simulink model "fuzzylogicMPPTmodified"  (R2024a)
settings: Solver=VariableStepAuto  StartTime=0.0  StopTime=20  RelTol=1e-3
undefined symbols (not defined in the file): Acid, Lead
libraries: spsSeriesRLCBranchLib x8, spsDiodeLib x4, spsBatteryLib x2, spsMosfetLib x2, spsPVArrayLib x2, fuzblock x1, spsPWMGeneratorDCDCLib x1, simulink x1, spsVoltageMeasurementLib x1, sps_lib x1
settings Model: Creator=Lenovo  LastModifiedBy=Lenovo

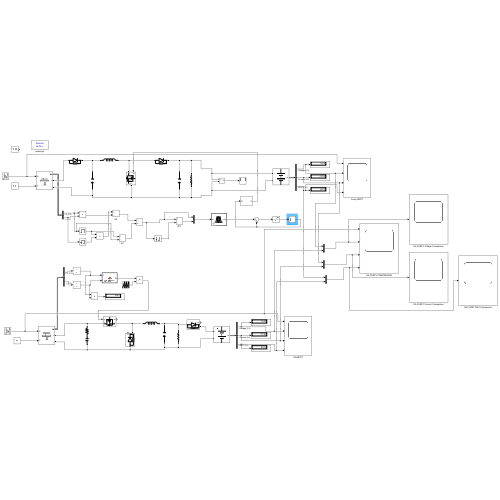
[thumbnail: Simulink's stored preview of the top-level diagram]
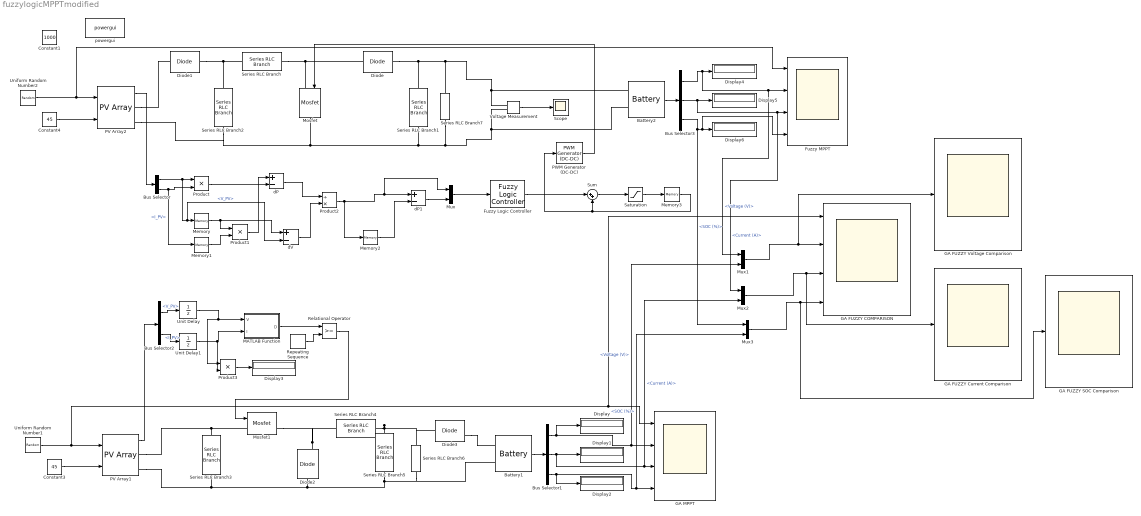
== system fuzzylogicMPPTmodified ==
  Battery1 : spsBatteryLib/Battery  BatType=Lead-Acid  ShowTempParam=off  ThermalPreset=no  ShowAgeParam=off  NomV=12  NomQ=40  SOC=60  Batt_Tr=0.1  PresetModel=on  MaxQ=41.6667  MinV=9  FullV=13.0658  Dis_rate=8  R=0.003  Normal_OP=12.4111  expZone="[12.2171     0.133333]"  current=[6.5 13 32.5]  Units=Time  Tci=20  NomT=20  T2=-30  MaxQ2=4.8  FullV2=7.1  Normal_OP2=5.655  expZone2="[6.58           1]"  Rca=0.6  ti=2000  Dp=0  Neq0=0  Tsim=1e6  Ta1=25  Qeol=5.4*0.9  Reol=0.013333*1.2  Char_age=[2.3478, 3]  Dis_age=[2.3478, 10]  N1=1500  N2=10500  N3=1000  N4=1400  Ta2=45  N5=950
  Battery2 : spsBatteryLib/Battery  BatType=Lead-Acid  ShowTempParam=off  ThermalPreset=no  ShowAgeParam=off  NomV=12  NomQ=40  SOC=60  Batt_Tr=0.1  PresetModel=on  MaxQ=41.6667  MinV=9  FullV=13.0658  Dis_rate=8  R=0.003  Normal_OP=12.4111  expZone="[12.2171     0.133333]"  current=[6.5 13 32.5]  Units=Time  Tci=20  NomT=20  T2=-30  MaxQ2=4.8  FullV2=7.1  Normal_OP2=5.655  expZone2="[6.58           1]"  Rca=0.6  ti=2000  Dp=0  Neq0=0  Tsim=1e6  Ta1=25  Qeol=5.4*0.9  Reol=0.013333*1.2  Char_age=[2.3478, 3]  Dis_age=[2.3478, 10]  N1=1500  N2=10500  N3=1000  N4=1400  Ta2=45  N5=950
  Bus Selector : BusSelector  OutputSignals=V_PV,I_PV
  Bus Selector1 : BusSelector  OutputSignals=Voltage (V),Current (A),SOC (%)
  Bus Selector2 : BusSelector  OutputSignals=V_PV,I_PV
  Bus Selector3 : BusSelector  OutputSignals=Voltage (V),Current (A),SOC (%)
  Constant1 : Constant  Value=1000
  Constant3 : Constant  Value=45
  Constant4 : Constant  Value=45
  Diode : spsDiodeLib/Diode  Ron=0.001  Lon=0  Vf=0.8  IC=0  UseSnubber=0  Rs=500  Cs=250e-9  Measurements=off
  Diode1 : spsDiodeLib/Diode  Ron=0.001  Lon=0  Vf=0.8  IC=0  UseSnubber=0  Rs=500  Cs=250e-9  Measurements=off
  Diode2 : spsDiodeLib/Diode  Ron=0.001  Lon=0  Vf=0.8  IC=0  UseSnubber=0  Rs=500  Cs=250e-9  Measurements=on
  Diode3 : spsDiodeLib/Diode  Ron=0.001  Lon=0  Vf=0.3  IC=0  UseSnubber=0  Rs=500  Cs=250e-9  Measurements=on
  Display{,1..6} (7 alike) : Display
  Fuzzy Logic Controller : fuzblock/Fuzzy Logic  Controller  FIS='pomppt.fis'  OutputSampleNumber=101  DataType=double  FuzzifiedInputs=off  RuleFiringStrengths=off  RuleOutputs=off  AggregatedOutputs=off  SimulateUsing=Interpreted execution  OutOfRangeInputValueMessage=warning  NoRuleFiredMessage=warning  EmptyOutputFuzzySetMessage=warning
  Fuzzy MPPT : Scope  NumInputPorts=4
  GA FUZZY COMPARISON : Scope  NumInputPorts=4
  GA FUZZY Current Comparison : Scope
  GA FUZZY SOC Comparison : Scope
  GA FUZZY Voltage Comparison : Scope
  GA MPPT : Scope  NumInputPorts=4
  MATLAB Function : MATLAB Function  TreatAsAtomicUnit=on
  Memory{,1..3} (4 alike) : Memory
  Mosfet : spsMosfetLib/Mosfet  Ron=0.1  Lon=0  Rd=0.01  Vfd=0  IC=0  Rs=1e5  Cs=inf  Measurements=off
  Mosfet1 : spsMosfetLib/Mosfet  Ron=0.1  Lon=0  Rd=0.01  Vfd=0  IC=0  Rs=1e5  Cs=inf  Measurements=on
  Mux{,1..3} (4 alike) : Mux  Inputs=2
  PV Array1 : spsPVArrayLib/PV Array  Npar=2  Nser=1  PlotType=array @ 1000 W/m2 & specified temperatures  S_vec="[ 1000  500  100 ]"  Temp_C_vec="[ 45 25  ]"  ModuleName=Lucky Power Technology LPS-6P6A-220-B  PlotWhenSelected=off  Pm=220.0599  Ncell=60  Voc=36.46  Isc=8.12  Vm=29.07  Im=7.57  beta_Voc_pc=-0.327  alpha_Isc_pc=0.051995  beta_Voc=-0.11922  alpha_Isc=0.004222  IL=8.1359  I0=8.141e-11  nI=0.93462  Rsh=211.4798  Rs=0.41331  RobustModel=off  RobustCellTemperature=313.3991  BAL=on  Tc=1e-6  Tfilter=5e-5
  PV Array2 : spsPVArrayLib/PV Array  Npar=2  Nser=1  PlotType=array @ 1000 W/m2 & specified temperatures  S_vec="[ 1000  500  100 ]"  Temp_C_vec="[ 45 25  ]"  ModuleName=Lucky Power Technology LPS-6P6A-220-B  PlotWhenSelected=off  Pm=220.0599  Ncell=60  Voc=36.46  Isc=8.12  Vm=29.07  Im=7.57  beta_Voc_pc=-0.327  alpha_Isc_pc=0.051995  beta_Voc=-0.11922  alpha_Isc=0.004222  IL=8.1359  I0=8.141e-11  nI=0.93462  Rsh=211.4798  Rs=0.41331  RobustModel=off  RobustCellTemperature=313.3991  BAL=on  Tc=1e-6  Tfilter=5e-5
  PWM Generator (DC-DC) : spsPWMGeneratorDCDCLib/PWM Generator (DC-DC)  Fsw=5000  Ts=0
  Product : Product
  Product1 : Product
  Product2 : Product  Inputs=/*
  Product3 : Product
  Relational Operator : RelationalOperator  OutDataTypeStr=boolean  RndMeth=Simplest  InputSameDT=off
  Repeating Sequence : simulink/Sources/Repeating Sequence  rep_seq_t=[0 0.0002]  rep_seq_y=[0 1]
  Saturation : Saturate
  Scope : Scope
  Series RLC Branch : spsSeriesRLCBranchLib/Series RLC Branch  LConnTagsString=__new0  RConnTagsString=__new0  BranchType=L  Resistance=1  Inductance=0.783e-2  SetiL0=off  InitialCurrent=0  Capacitance=1e-6  Setx0=off  InitialVoltage=0  Measurements=None
  Series RLC Branch1 : spsSeriesRLCBranchLib/Series RLC Branch  LConnTagsString=__new0  RConnTagsString=__new0  BranchType=C  Resistance=1  Inductance=50e-6  SetiL0=off  InitialCurrent=0  Capacitance=50e-6  Setx0=off  InitialVoltage=0  Measurements=None
  Series RLC Branch2 : spsSeriesRLCBranchLib/Series RLC Branch  LConnTagsString=__new0  RConnTagsString=__new0  BranchType=C  Resistance=1  Inductance=50e-6  SetiL0=off  InitialCurrent=0  Capacitance=4000e-6  Setx0=off  InitialVoltage=0  Measurements=None
  Series RLC Branch3 : spsSeriesRLCBranchLib/Series RLC Branch  LConnTagsString=__new0  RConnTagsString=__new0  BranchType=RC  Resistance=0.0001  Inductance=1e-3  SetiL0=off  InitialCurrent=0  Capacitance=1000e-6  Setx0=off  InitialVoltage=0  Measurements=None
  Series RLC Branch4 : spsSeriesRLCBranchLib/Series RLC Branch  LConnTagsString=__new0  RConnTagsString=__new0  BranchType=L  Resistance=1  Inductance=0.783e-2  SetiL0=off  InitialCurrent=0  Capacitance=1e-6  Setx0=off  InitialVoltage=0  Measurements=None
  Series RLC Branch5 : spsSeriesRLCBranchLib/Series RLC Branch  LConnTagsString=__new0  RConnTagsString=__new0  BranchType=C  Resistance=1  Inductance=1e-3  SetiL0=off  InitialCurrent=0  Capacitance=364e-6  Setx0=off  InitialVoltage=0  Measurements=None
  Series RLC Branch6 : spsSeriesRLCBranchLib/Series RLC Branch  LConnTagsString=__new0  RConnTagsString=__new0  BranchType=R  Resistance=4  Inductance=1e-3  SetiL0=off  InitialCurrent=0  Capacitance=1e-6  Setx0=off  InitialVoltage=0  Measurements=Branch voltage and current
  Series RLC Branch7 : spsSeriesRLCBranchLib/Series RLC Branch  LConnTagsString=__new0  RConnTagsString=__new0  BranchType=R  Resistance=4  Inductance=1e-3  SetiL0=off  InitialCurrent=0  Capacitance=1e-6  Setx0=off  InitialVoltage=0  Measurements=Branch voltage and current
  Sum : Sum  Inputs=|++
  Uniform Random Number1 : UniformRandomNumber  Minimum=20  Maximum=1000  Seed=342  SampleTime=1
  Uniform Random Number2 : UniformRandomNumber  Minimum=20  Maximum=1000  Seed=342  SampleTime=1
  Unit Delay : UnitDelay  SampleTime=1e-4  HasFrameUpgradeWarning=on
  Unit Delay1 : UnitDelay  SampleTime=1e-4  HasFrameUpgradeWarning=on
  Voltage Measurement : spsVoltageMeasurementLib/Voltage Measurement  PhasorSimulation=off  OutputType=Complex  PSBequivalent=0
  dP : Sum  Inputs=+-
  dP1 : Sum  Inputs=+-
  dV : Sum  Inputs=+-
  powergui : sps_lib/powergui  Priority=1  SimulationMode=Discrete  SampleTime=50e-6  frequency=60  Iterations=50  frequencyindice=0  Pbase=100e6  ErrMax=1e-4  UnitsV=kV  UnitsW=MW  buscounter=0  FunctionMessages=off  echomessages=off  EnableUseOfTLC=off  CurrentSourceSwitches=off  DisableSnubberDevices=off  DisableRonSwitches=off  DisableVfSwitches=off  DisplayEquations=off  AutomaticDiscreteSolvers=off  SolverType=Tustin/Backward Euler (TBE)  Interpol=off  ExternalGateDelay=off  methode=off  Ts=100  x0status=blocks  SPID=on  SwTol=0  HookPort=off  NonlinearTolerance=1e-4  nMaxIteration=100  ContinueOnMaxIteration=off  RestoreLinks=warning  ResistiveCurrentMeasurement=off  Frange=[0:2:500]  Ylog=off  Xlog=on  ShowGrid=off  save=off  variable=ZData  structure=0  ZoomFFT=off  StartTime=0.0  cycles=1  DisplayStyle=1  fundamental=60  FreqAxis=off  MaxFrequency=1000  frequencyindicesteady=1  RmsSteady=1  display=off
  wires:
  PV Array2/1 -> Bus Selector/1
  Bus Selector/1 -> dV/2, Memory/1, Product/1  "<V_PV>"
  Bus Selector/2 -> Memory1/1, Product/2  "<I_PV>"
  Product/1 -> dP/2
  Memory/1 -> dV/1, Product1/1
  Memory1/1 -> Product1/2
  Product1/1 -> dP/1
  dP/1 -> Product2/1
  dV/1 -> Product2/2
  Product2/1 -> Memory2/1, Mux/1, dP1/1
  Memory2/1 -> dP1/2
  dP1/1 -> Mux/2
  Mux/1 -> Fuzzy Logic Controller/1
  Sum/1 -> Saturation/1
  Saturation/1 -> Memory3/1
  Memory3/1 -> Sum/2, PWM Generator (DC-DC)/1
  Fuzzy Logic Controller/1 -> Sum/1
  PWM Generator (DC-DC)/1 -> Mosfet/1
  Voltage Measurement/1 -> Scope/1
  Product3/1 -> Display3/1
  PV Array1/1 -> Bus Selector2/1
  Unit Delay/1 -> Product3/1, MATLAB Function/1(V)
  Bus Selector1/1 -> Mux1/2, GA MPPT/2, Display/1  "<Voltage (V)>"
  Bus Selector2/2 -> Unit Delay1/1  "<I_PV>"
  Uniform Random Number1/1 -> GA FUZZY COMPARISON/1, GA MPPT/1, PV Array1/1
  Repeating Sequence/1 -> Relational Operator/2
  Bus Selector1/2 -> Mux2/2, GA MPPT/3, Display1/1  "<Current (A)>"
  Bus Selector1/3 -> Mux3/2, GA MPPT/4, Display2/1  "<SOC (%)>"
  MATLAB Function/1(D) -> Relational Operator/1
  Relational Operator/1 -> Mosfet1/1
  Unit Delay1/1 -> Product3/2, MATLAB Function/2(I)
  Bus Selector2/1 -> Unit Delay/1  "<V_PV>"
  Battery1/1 -> Bus Selector1/1
  Constant3/1 -> PV Array1/2
  Uniform Random Number2/1 -> Fuzzy MPPT/1, PV Array2/1
  Constant4/1 -> PV Array2/2
  Bus Selector3/2 -> Mux2/1, Fuzzy MPPT/3, Display5/1  "<Current (A)>"
  Bus Selector3/3 -> Mux3/1, Fuzzy MPPT/4, Display6/1  "<SOC (%)>"
  Battery2/1 -> Bus Selector3/1
  Bus Selector3/1 -> Mux1/1, Fuzzy MPPT/2, Display4/1  "<Voltage (V)>"
  Mux1/1 -> GA FUZZY Voltage Comparison/1, GA FUZZY COMPARISON/2
  Mux2/1 -> GA FUZZY Current Comparison/1, GA FUZZY COMPARISON/3
  Mux3/1 -> GA FUZZY SOC Comparison/1, GA FUZZY COMPARISON/4
  connections:
  Series RLC Branch/LConn1 -- Diode1/RConn1 -- Series RLC Branch2/LConn1
  Series RLC Branch/RConn1 -- Diode/LConn1 -- Mosfet/LConn1
  Diode/RConn1 -- Series RLC Branch1/LConn1 -- Battery2/LConn1 -- Voltage Measurement/LConn1 -- Series RLC Branch7/LConn1
  Voltage Measurement/LConn2 -- Series RLC Branch7/RConn1 -- Series RLC Branch1/RConn1 -- PV Array2/RConn2 -- Series RLC Branch2/RConn1 -- Mosfet/RConn1 -- Battery2/LConn2
  PV Array2/RConn1 -- Diode1/LConn1
  Series RLC Branch5/RConn1 -- PV Array1/RConn2 -- Series RLC Branch3/RConn1 -- Diode2/LConn1 -- Series RLC Branch6/RConn1 -- Battery1/LConn2
  Series RLC Branch3/LConn1 -- PV Array1/RConn1 -- Mosfet1/LConn1
  Series RLC Branch5/LConn1 -- Series RLC Branch4/RConn1 -- Series RLC Branch6/LConn1 -- Diode3/LConn1
  Diode2/RConn1 -- Mosfet1/RConn1 -- Series RLC Branch4/LConn1
  Diode3/RConn1 -- Battery1/LConn1

== matlab function fuzzylogicMPPTmodified/MATLAB Function ==
  data: V input; D output; I input
function D = GA_MPPT(V, I)
%#codegen
% GA_MPPT - Maximum Power Point Tracking using Genetic Algorithm
% Input: V (tegangan), I (arus)
% Output: D (duty cycle optimal, skalar double)

persistent Population Fitness Elite Pop_size Max_iterations t ...
    pc pm LB UB dim convergence_count prev_best last_D

% Deklarasikan ukuran maksimum untuk variabel persisten
coder.varsize('Population', [100, 1], [1 0]);
coder.varsize('Fitness', [100, 1], [1 0]);

% Inisialisasi nilai default untuk last_D jika belum ada
if isempty(last_D)
    last_D = 0.5;
end

if isempty(Population)
    %% Inisialisasi Parameter GA
    Pop_size = 20;          % Ukuran populasi
    Max_iterations = 50;    % Maksimum iterasi dalam satu siklus GA
    dim = 1;                % Dimensi masalah (1D: duty cycle)
    LB = 0.05;              % Batas bawah duty cycle
    UB = 0.95;              % Batas atas duty cycle
    
    % Parameter GA
    pc = 0.8;               % Probabilitas crossover
    pm = 0.1;               % Probabilitas mutasi
    
    % Inisialisasi populasi awal secara acak dalam rentang [LB, UB]
    Population = LB + (UB - LB) .* rand(Pop_size, dim);
    
    % Evaluasi fitness awal
    Fitness = zeros(Pop_size, 1);
    for i = 1:Pop_size
        Fitness(i) = getPowerForD(Population(i), V, I);
    end
    
    % Tentukan solusi elite awal
    [~, idx] = max(Fitness);
    Elite = Population(idx, :);
    t = 1;
    convergence_count = 0;
    prev_best = Elite;
    last_D = Elite(1);
end

%% Evaluasi populasi saat ini
for i = 1:Pop_size
    Fitness(i) = getPowerForD(Population(i), V, I);
end

% Update elite berdasarkan evaluasi terbaru
[~, elite_idx] = max(Fitness);
current_elite = Population(elite_idx, :);
current_elite_fitness = Fitness(elite_idx);
if current_elite_fitness > getPowerForD(Elite(1), V, I)
    Elite = current_elite;
end

%% Seleksi Orang Tua menggunakan Tournament Selection (ukuran tournament = 2)
parent_indices = zeros(Pop_size, 1);
for i = 1:Pop_size
    candidates = randperm(Pop_size, 2);
    if Fitness(candidates(1)) > Fitness(candidates(2))
        parent_indices(i) = candidates(1);
    else
        parent_indices(i) = candidates(2);
    end
end

%% Crossover - BLX-α (untuk nilai kontinu)
Offspring = zeros(Pop_size, dim);
for i = 1:2:(Pop_size - 1)
    p1 = Population(parent_indices(i), :);
    p2 = Population(parent_indices(i+1), :);
    
    if rand() < pc
        alpha_val = 0.5;   % Parameter BLX-alpha
        d = abs(p1 - p2);
        lower_bound = min(p1, p2) - alpha_val * d;
        upper_bound = max(p1, p2) + alpha_val * d;
        % Pastikan nilai dalam rentang [LB, UB]
        lower_bound = max(lower_bound, LB);
        upper_bound = min(upper_bound, UB);
        Offspring(i,:) = lower_bound + (upper_bound - lower_bound) * rand();
        Offspring(i+1,:) = lower_bound + (upper_bound - lower_bound) * rand();
    else
        Offspring(i,:) = p1;
        Offspring(i+1,:) = p2;
    end
end

%% Mutasi - Non-uniform mutation berdasarkan iterasi
for i = 1:Pop_size
    if rand() < pm
        % Nilai tau mengecil seiring bertambahnya iterasi
        tau = (1 - t / Max_iterations)^2;
        if rand() < 0.5
            Offspring(i) = Offspring(i) + (UB - Offspring(i)) * tau * randn();
        else
            Offspring(i) = Offspring(i) - (Offspring(i) - LB) * tau * randn();
        end
    end
end

% Batasi nilai offspring agar tetap berada di [LB, UB]
Offspring = min(max(Offspring, LB), UB);

%% Evaluasi Fitness Offspring
OffspringFitness = zeros(Pop_size, 1);
for i = 1:Pop_size
    OffspringFitness(i) = getPowerForD(Offspring(i), V, I);
end

%% Replacement dengan Elitism
CombinedPop = [Population; Offspring];
CombinedFitness = [Fitness; OffspringFitness];
[sortedFitness, sortIdx] = sort(CombinedFitness, 'descend');
NewPopulation = CombinedPop(sortIdx(1:Pop_size), :);
NewFitness = sortedFitness(1:Pop_size);

Population = NewPopulation;
Fitness = NewFitness;

% Update Elite berdasarkan populasi baru
[~, new_elite_idx] = max(Fitness);
Elite = Population(new_elite_idx, :);
D = Elite(1);
last_D = D;

%% Cek Konvergensi: Periksa jika perubahan elite sangat kecil
if abs(prev_best - Elite) < 0.005
    convergence_count = convergence_count + 1;
else
    convergence_count = 0;
end
prev_best = Elite;

%% Update Counter Iterasi (generasi)
if t >= Max_iterations || convergence_count >= 5
    % Alih-alih reset penuh, pertahankan 50% populasi terbaik dan isi sisanya secara acak
    t = 1;
    convergence_count = 0;
    [~, sortIdx] = sort(Fitness, 'descend');
    ElitePop = Population(sortIdx(1:floor(Pop_size/2)), :); % Pertahankan 50% terbaik
    RandomPop = LB + (UB - LB) .* rand(Pop_size - floor(Pop_size/2), dim);
    Population = [ElitePop; RandomPop];
    for i = 1:Pop_size
        Fitness(i) = getPowerForD(Population(i), V, I);
    end
else
    t = t + 1;
end

% Pastikan output duty cycle berada di dalam batas [LB, UB]
if isempty(D) || isnan(D)
    D = last_D;
else
    D = max(min(D, UB), LB);
end

end

%% Fungsi Evaluasi Daya
function P = getPowerForD(D, V, I)
    % Menghitung daya berdasarkan D, V, dan I
    % Asumsi sederhana: P = V * I * f(D), dengan f(D) adalah fungsi kuadrat
    % Dalam praktik, ganti dengan model nyata dari sistem PV dan konverter
    P = V * I * (-(D - 0.5)^2 + 1); % Maksimum di D = 0.5 untuk demonstrasi
end
